simulink model "sys"  (R2017a)
settings: Solver=FixedStepAuto  StartTime=0.0  StopTime=40  FixedStep=0.02  RelTol=1e-3
values from neighbouring files (symbols this model uses):
  Fm1 = [0 1;0 0]    [OBS_CONT.m]
  Fm2 = [0 1;-(km2)/(jm2) -(bm2)/(jm2)]    [OBS_CONT.m]
  Gm1 = [0;1/(jm1)]    [OBS_CONT.m]
  Gm2 = [0;1/(jm2)]    [OBS_CONT.m]
  Kc_m1 = place(Fm1,Gm1,pc_m1)    [OBS_CONT.m]
  Kc_m2 = place(Fm2,Gm2,pc_m2)    [OBS_CONT.m]
  Kr_m1 = rscale(Fm1,Gm1,Hm1,Dm1,Kc_m1)    [OBS_CONT.m]
  Kr_m2 = rscale(Fm2,Gm2,Hm2,Dm2,Kc_m2)    [OBS_CONT.m]
settings Model: Creator=ASUS  LastModifiedBy=ASUS

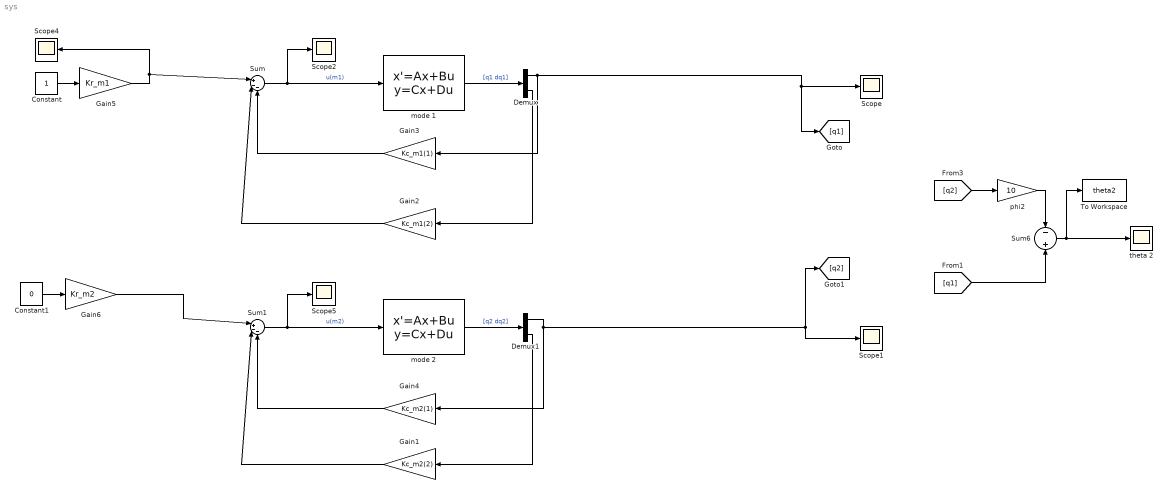
== system sys ==
  Constant : Constant
  Constant1 : Constant  Value=0
  Demux : Demux  Outputs=2
  Demux1 : Demux  Outputs=2
  Gain1 : Gain  Gain=Kc_m2(2)
  Gain2 : Gain  Gain=Kc_m1(2)
  Gain3 : Gain  Gain=Kc_m1(1)
  Gain4 : Gain  Gain=Kc_m2(1)
  Gain5 : Gain  Gain=Kr_m1
  Gain6 : Gain  Gain=Kr_m2
  Scope{,1..2,4..5} (5 alike) : Scope
  Sum : Sum  Inputs=|+--
  Sum1 : Sum  Inputs=|+--
  Sum6 : Sum  Inputs=-+
  To Workspace : ToWorkspace  VariableName=theta2  SaveFormat=Timeseries  SampleTime=-1
  mode 1 : StateSpace  A=Fm1  B=Gm1  C=[1 0;0 1]  D=[0;0]  X0=0
  mode 2 : StateSpace  A=Fm2  B=Gm2  C=[1 0;0 1]  D=[0;0]  X0=0
  "phi2 " : Gain  Gain=10
  theta 2 : Scope
  wires:
  Sum/1 -> Scope2/1, mode 1/1  "u(m1)"
  mode 1/1 -> Demux/1  "[q1 dq1]"
  Sum1/1 -> Scope5/1, mode 2/1  "u(m2)"
  Gain2/1 -> Sum/2
  Gain1/1 -> Sum1/2
  Demux/1 -> [q1], Scope/1, Gain3/1
  Gain3/1 -> Sum/3
  Demux/2 -> Gain2/1
  Demux1/1 -> Scope1/1, [q2], Gain4/1
  Demux1/2 -> Gain1/1
  mode 2/1 -> Demux1/1  "[q2 dq2]"
  Gain4/1 -> Sum1/3
  [q2] -> "phi2 "/1
  [q1] -> Sum6/2
  "phi2 "/1 -> Sum6/1
  Sum6/1 -> To Workspace/1, theta 2/1
  Constant/1 -> Gain5/1
  Constant1/1 -> Gain6/1
  Gain5/1 -> Sum/1, Scope4/1
  Gain6/1 -> Sum1/1
